simulink library "EmE_MBD_Blockset"  (R2018a)
settings: Solver=ode1  StartTime=0.0  StopTime=Inf  FixedStep=0.001  RelTol=1e-3  EnableMultiTasking=on
PostLoadFcn:
  | , if any(exist('dsrtsu_mdlpostloadfcn', 'file') == [2, 3, 6]), try dsrtsu_mdlpostloadfcn('Execute', bdroot); catch fprintf('Error in PostLoadFcn (dsrtsu_mdlpostloadfcn) for model "%s":\n %s\n', bdroot, lasterr); end, end,
undefined symbols (not defined in the file or in its folder): ENUM_TSC1_CONTROL_PURPOSE_T, gcbh, GLB_SWITCH_T
libraries: simulink x237, $bdroot x115, simulink_need_slupdate x26, MotoHawk_lib x13, simulink_extras x3
(part 3 of 11)

== system EmE_MBD_Blockset/Sources ==
  In : Inport
  APV : Constant  Value=0  mask(Constant APV (EmE)){conval=0}
      mask prompts: conval "Tunable parameter:"
      mask help: Generate a tunable parameter value (configuration or calibration).
      mask init:
      | set_param(gcbh,'Value',conval)
  CPV : Constant  Value=0  mask(Constant CPV (EmE)){conval=0}
      mask prompts: conval "Constant value:"
      mask help: Generate a constant value.
      mask init:
      | set_param(gcbh,'Value',conval)
      mask DialogControl DescTextVar Prompt: Constant parameter value.
  Digital Clock : DigitalClock  SampleTime=-1
  Ground : Ground
  dT : Subsystem  mask(Delta time (dT) (EmE)){}
      mask help: This block calculates a "delta time" or execution rate of a subsystem.
      mask init:
      | alpha=0:2*pi/100:2*pi;
      mask Display:
      | plot(0.3+0.15*cos(alpha),0.5+0.4*sin(alpha));
      | plot([0.3 0.3 0.4],[0.7 0.5 0.5]);
      | fprintf('              dT');

== system EmE_MBD_Blockset/User-Defined Functions ==
  Compare_VIN_data : Subsystem
  Determine_engine_speed_from_vehicle_speed : Subsystem
  Determine_permanent_magnet_motor_BEMF_volts_at_magnet_temp : Subsystem
  Determine_vehicle_speed_from_trans_output_shaft_speed : Subsystem
  Latching_mutual_exclusion : Subsystem
  Snoop : Subsystem  mask(CCP_Snoop){setup=off, a2l=DC4_A1519R191A_modified_checksum.a2l, frstPID=64, sizeDAQ=16, name1=CA_Ambient_air_temp_value, name2=Air_temp_post_int.Value, name3=CPM_Crank_power, name4=CA_Vehicle_speed, name5=CA_Ecfan_fspd_value, name6=CPM_Air_temp_pre_int, name7=AMF_Fresh_air, name8=CA_Ambient_air_press_value, name9=CA_Engine_speed, name10=CA_Cool_temp_value, name11=CREC_Eng_run_time_since_key_on, name12=F_CPM_Int_enabled, address1=400076EC, address2=00501F12, address3=4000C33C, address4=40007564, address5=40007D66, address6=4000C33A, address7=4000BF4A, address8=4000768C, address9=40007530, address10=4000750C, address11=40006210, address12=4000C324, type1=single, type2=uint16, type3=int16, type4=single, type5=uint16, type6=uint16, type7=uint16, type8=single, type9=single, type10=single, type11=uint32, type12=uint8, convert1=[1  1  0], convert2=[1  10   0], convert3=[1  10   0], convert4=[1  1  0], convert5=[1  1  0], convert6=[1  10   0], convert7=[1  40   0], convert8=[1  1  0], convert9=[1  1  0], convert10=[1  1  0], convert11=[1  1  0], convert12=[1  1  0], default1=0, default2=0, default3=0, default4=0, default5=0, default6=0, default7=0, default8=0, default9=0, default10=0, default11=0, default12=0}
      mask prompts: setup "Check to launch auto setup"; a2l "SoftwareA2L"; frstPID "First PID (as dec)"; sizeDAQ "DAQ Length (as dec)"; name1 "Signal Name"; name2 "Signal Name"; name3 "Signal Name"; name4 "Signal Name"; name5 "Signal Name"; name6 "Signal Name"; name7 "Signal Name"; name8 "Signal Name"; name9 "Signal Name"; name10 "Signal Name"; name11 "Signal Name"; name12 "Signal Name"; address1 "Memory Address"; address2 "Memory Address"; address3 "Memory Address"; address4 "Memory Address"; address5 "Memory Address"; address6 "Memory Address"; address7 "Memory Address"; address8 "Memory Address"; address9 "Memory Address"; address10 "Memory Address"; address11 "Memory Address"; address12 "Memory Address"; type1 "Data Type"; type2 "Data Type"; type3 "Data Type"; type4 "Data Type"; type5 "Data Type"; type6 "Data Type"; type7 "Data Type"; type8 "Data Type"; type9 "Data Type"; type10 "Data Type"; type11 "Data Type"; type12 "Data Type"; convert1 "Signal conversion vector [A B C] :: (A/B) * x + C"; convert2 "Signal conversion vector [A B C] :: (A/B) * x + C"; convert3 "Signal conversion vector [A B C] :: (A/B) * x + C"; convert4 "Signal conversion vector [A B C] :: (A/B) * x + C"; convert5 "Signal conversion vector [A B C] :: (A/B) * x + C"; convert6 "Signal conversion vector [A B C] :: (A/B) * x + C"; convert7 "Signal conversion vector [A B C] :: (A/B) * x + C"; convert8 "Signal conversion vector [A B C] :: (A/B) * x + C"; convert9 "Signal conversion vector [A B C] :: (A/B) * x + C"; convert10 "Signal conversion vector [A B C] :: (A/B) * x + C"; convert11 "Signal conversion vector [A B C] :: (A/B) * x + C"; convert12 "Signal conversion vector [A B C] :: (A/B) * x + C"; default1 "Default Value"; default2 "Default Value"; default3 "Default Value"; default4 "Default Value"; default5 "Default Value"; default6 "Default Value"; default7 "Default Value"; default8 "Default Value"; default9 "Default Value"; default10 "Default Value"; default11 "Default Value"; default12 "Default Value"
      mask init:
      | CCP_Snoop_init
      mask Callback setup: snoop_cfg(gcbh)
      mask TypeOptions type1: uint8 | int8 | uint16 | int16 | uint32 | int32 | single
      mask TypeOptions type2: uint8 | int8 | uint16 | int16 | uint32 | int32 | single
      mask TypeOptions type3: uint8 | int8 | uint16 | int16 | uint32 | int32 | single
      mask TypeOptions type4: uint8 | int8 | uint16 | int16 | uint32 | int32 | single
      mask TypeOptions type5: uint8 | int8 | uint16 | int16 | uint32 | int32 | single
      mask TypeOptions type6: uint8 | int8 | uint16 | int16 | uint32 | int32 | single
      mask TypeOptions type7: uint8 | int8 | uint16 | int16 | uint32 | int32 | single
      mask TypeOptions type8: uint8 | int8 | uint16 | int16 | uint32 | int32 | single
      mask TypeOptions type9: uint8 | int8 | uint16 | int16 | uint32 | int32 | single
      mask TypeOptions type10: uint8 | int8 | uint16 | int16 | uint32 | int32 | single
      mask TypeOptions type11: uint8 | int8 | uint16 | int16 | uint32 | int32 | single
      mask TypeOptions type12: uint8 | int8 | uint16 | int16 | uint32 | int32 | single
      mask DialogControl ParameterTabVar0 Prompt: Setup
      mask DialogControl ParameterTabVar01 Prompt: Signal1
      mask DialogControl ParameterTabVar012 Prompt: Signal2
      mask DialogControl ParameterTabVar0123 Prompt: Signal3
      mask DialogControl ParameterTabVar01234 Prompt: Signal4
      mask DialogControl ParameterTabVar012345 Prompt: Signal5
      mask DialogControl ParameterTabVar0123456 Prompt: Signal6
      mask DialogControl ParameterTabVar01234567 Prompt: Signal7
      mask DialogControl ParameterTabVar012345678 Prompt: Signal8
      mask DialogControl ParameterTabVar0123456789 Prompt: Signal9
      mask DialogControl ParameterTabVar012345678910 Prompt: Signal10
      mask DialogControl ParameterTabVar01234567891011 Prompt: Signal11
      mask DialogControl ParameterTabVar0123456789101112 Prompt: Signal12
      mask Display:
      | image(imread('snoop.jpg'))
      | % port_label('output',1,'Data')
      | text(.021,.95,a2lFile,'horizontalAlign', 'left')
      | text(1,0.5,sigDisp,'horizontalAlign', 'right')
  TRUCK_1841_VIN_CPV : Constant  Value=uint8('2NKHHM7X5JM216659')
  wires:
  TRUCK_1841_VIN_CPV/1 -> Compare_VIN_data/1(VIN_Input_uint8)

== system EmE_MBD_Blockset/Controllers/Generic_PID_Governor_3 ==
  F_GPID_reset : Inport
  GPID_setpoint : Inport  Port=2
  GPID_feedback : Inport  Port=3
  GPID_actual_system_output : Inport  Port=4
  GPID_slew_init : Inport  Port=5
  GPID_feed_forward : Inport  Port=6
  GPID_slew_inc_setpoint : Inport  Port=7
  GPID_slew_dec_setpoint : Inport  Port=8
  GPID_output_max : Inport  Port=9
  GPID_output_min : Inport  Port=10
  GPID_Kp : Inport  Port=11
  GPID_Ki : Inport  Port=12
  GPID_Kd : Inport  Port=13
  GPID_T_filt_d : Inport  Port=14
  GPID_T_filt_control_error : Inport  Port=15
  F_GPID_aw_cond_integration : Inport  Port=16
  GPID_aw_hysteresis : Inport  Port=17
  GPID_dT : Inport  Port=18
  F_GPID_aw_hold_i_term : Inport  Port=19
  Calculate_PID_terms : Subsystem
  Determine_control_error : Subsystem
  Output_PID : Subsystem
  Reset_governor : Subsystem
  Unit_Delay : UnitDelay  SampleTime=-1
      settings: AttributesFormatString=IC: %<vinit>
  GPID_output : Outport
  GPID_output_unlim : Outport  Port=2
  GPID_control_error : Outport  Port=3
  GPID_p_term : Outport  Port=4
  GPID_i_term : Outport  Port=5
  GPID_d_term : Outport  Port=6
  F_GPID_hold_i_term : Outport  Port=7
  wires:
  Output_PID/2(GPID_output_unlim) -> GPID_output_unlim/1, Unit_Delay/1
  Calculate_PID_terms/1(GPID_p_term) -> Output_PID/1(GPID_p_term), GPID_p_term/1
  F_GPID_aw_hold_i_term/1 -> Calculate_PID_terms/12(F_GPID_aw_hold_i_term)
  GPID_aw_hysteresis/1 -> Calculate_PID_terms/11(GPID_aw_hysteresis)
  F_GPID_aw_cond_integration/1 -> Calculate_PID_terms/10(F_GPID_aw_cond_integration)
  GPID_feed_forward/1 -> Output_PID/6(GPID_feed_forward), Calculate_PID_terms/5(GPID_feed_forward)
  GPID_actual_system_output/1 -> Calculate_PID_terms/4(GPID_actual_system_output)
  GPID_output_min/1 -> Output_PID/4(GPID_output_min)
  GPID_output_max/1 -> Output_PID/5(GPID_output_max)
  GPID_Kd/1 -> Calculate_PID_terms/8(GPID_Kd)
  GPID_Ki/1 -> Calculate_PID_terms/7(GPID_Ki)
  GPID_feedback/1 -> Determine_control_error/7(GPID_feedback)
  GPID_slew_dec_setpoint/1 -> Determine_control_error/5(GPID_slew_dec_setpoint)
  GPID_setpoint/1 -> Determine_control_error/3(GPID_setpoint)
  GPID_slew_init/1 -> Determine_control_error/2(GPID_slew_init)
  F_GPID_reset/1 -> Reset_governor/1(F_GPID_reset)
  Calculate_PID_terms/4(F_GPID_hold_i_term) -> F_GPID_hold_i_term/1
  Calculate_PID_terms/3(GPID_d_term) -> Output_PID/3(GPID_d_term), GPID_d_term/1
  GPID_T_filt_control_error/1 -> Determine_control_error/8(GPID_T_filt_control_error)
  Reset_governor/1(F_GPID_reset_gov) -> Determine_control_error/1(F_GPID_reset_gov), Calculate_PID_terms/1(F_GPID_reset_gov)
  GPID_slew_inc_setpoint/1 -> Determine_control_error/4(GPID_slew_inc_setpoint)
  GPID_Kp/1 -> Calculate_PID_terms/6(GPID_Kp)
  Determine_control_error/1(GPID_control_error) -> Calculate_PID_terms/2(GPID_control_error), GPID_control_error/1
  Calculate_PID_terms/2(GPID_i_term) -> Output_PID/2(GPID_i_term), GPID_i_term/1
  GPID_T_filt_d/1 -> Calculate_PID_terms/9(GPID_T_filt_d)
  GPID_dT/1 -> Determine_control_error/6(GPID_dT), Calculate_PID_terms/3(GPID_dT)
  Unit_Delay/1 -> Calculate_PID_terms/13(GPID_output_unlim_prev)
  Output_PID/1(GPID_output) -> GPID_output/1

== system EmE_MBD_Blockset/Controllers/Generic_PID_Governor_4 ==
  F_GPID_reset : Inport
  GPID_setpoint : Inport  Port=2
  GPID_feedback : Inport  Port=3
  GPID_actual_system_output : Inport  Port=4
  GPID_slew_init : Inport  Port=5
  GPID_feed_forward : Inport  Port=6
  GPID_slew_inc_setpoint : Inport  Port=7
  GPID_slew_dec_setpoint : Inport  Port=8
  GPID_output_max : Inport  Port=9
  GPID_output_min : Inport  Port=10
  GPID_Kp : Inport  Port=11
  GPID_Ki : Inport  Port=12
  GPID_Kd : Inport  Port=13
  GPID_T_filt_d : Inport  Port=14
  GPID_T_filt_control_error : Inport  Port=15
  F_GPID_aw_cond_integration : Inport  Port=16
  GPID_aw_hysteresis : Inport  Port=17
  GPID_dT : Inport  Port=18
  F_GPID_aw_hold_i_term : Inport  Port=19
  Calculate_PID_terms : Subsystem
  Determine_control_error : Subsystem
  Output_PID : Subsystem
  Reset_governor : Subsystem
  Unit_Delay : UnitDelay  SampleTime=-1
      settings: AttributesFormatString=IC: %<vinit>
  Unit_Delay1 : UnitDelay  SampleTime=-1
      settings: AttributesFormatString=IC: %<vinit>
  GPID_output : Outport
  GPID_output_unlim : Outport  Port=2
  GPID_control_error : Outport  Port=3
  GPID_p_term : Outport  Port=4
  GPID_i_term : Outport  Port=5
  GPID_d_term : Outport  Port=6
  F_GPID_hold_i_term : Outport  Port=7
  wires:
  F_GPID_reset/1 -> Reset_governor/1(F_GPID_reset)
  Reset_governor/1(F_GPID_reset_gov) -> Calculate_PID_terms/1(F_GPID_reset_gov), Determine_control_error/1(F_GPID_reset_gov)
  GPID_slew_init/1 -> Determine_control_error/2(GPID_slew_init)
  GPID_setpoint/1 -> Determine_control_error/3(GPID_setpoint)
  GPID_slew_inc_setpoint/1 -> Determine_control_error/4(GPID_slew_inc_setpoint)
  GPID_slew_dec_setpoint/1 -> Determine_control_error/5(GPID_slew_dec_setpoint)
  GPID_feedback/1 -> Determine_control_error/7(GPID_feedback)
  GPID_T_filt_control_error/1 -> Determine_control_error/8(GPID_T_filt_control_error)
  Determine_control_error/1(GPID_control_error) -> GPID_control_error/1, Calculate_PID_terms/2(GPID_control_error)
  GPID_actual_system_output/1 -> Calculate_PID_terms/4(GPID_actual_system_output)
  GPID_feed_forward/1 -> Output_PID/6(GPID_feed_forward), Calculate_PID_terms/5(GPID_feed_forward)
  GPID_Kp/1 -> Calculate_PID_terms/6(GPID_Kp)
  GPID_Ki/1 -> Calculate_PID_terms/7(GPID_Ki)
  GPID_Kd/1 -> Calculate_PID_terms/8(GPID_Kd)
  GPID_T_filt_d/1 -> Calculate_PID_terms/9(GPID_T_filt_d)
  F_GPID_aw_cond_integration/1 -> Calculate_PID_terms/10(F_GPID_aw_cond_integration)
  GPID_aw_hysteresis/1 -> Calculate_PID_terms/11(GPID_aw_hysteresis)
  GPID_dT/1 -> Determine_control_error/6(GPID_dT), Calculate_PID_terms/3(GPID_dT)
  F_GPID_aw_hold_i_term/1 -> Calculate_PID_terms/12(F_GPID_aw_hold_i_term)
  Calculate_PID_terms/1(GPID_p_term) -> Output_PID/1(GPID_p_term), GPID_p_term/1
  Calculate_PID_terms/2(GPID_i_term) -> Output_PID/2(GPID_i_term), GPID_i_term/1
  Calculate_PID_terms/3(GPID_d_term) -> GPID_d_term/1, Output_PID/3(GPID_d_term)
  Calculate_PID_terms/4(F_GPID_hold_i_term) -> F_GPID_hold_i_term/1
  Unit_Delay/1 -> Calculate_PID_terms/13(GPID_output_unlim_prev)
  GPID_output_max/1 -> Output_PID/5(GPID_output_max)
  GPID_output_min/1 -> Output_PID/4(GPID_output_min)
  Output_PID/1(GPID_output) -> GPID_output/1
  Output_PID/2(GPID_output_unlim) -> GPID_output_unlim/1, Unit_Delay/1
  Unit_Delay1/1 -> Calculate_PID_terms/14(GPID_output_delta)
  Output_PID/3(GPID_output_delta) -> Unit_Delay1/1

== system EmE_MBD_Blockset/Controllers/PID_saturating_terms ==
  Setpoint : Inport
  Feedback : Inport  Port=2
  Feedforward : Inport  Port=3
  Kp : Inport  Port=4
  Ki : Inport  Port=5
  Kd : Inport  Port=6
  Kff : Inport  Port=7
  Kfb : Inport  Port=8
  dT : Inport  Port=9
  P_min : Inport  Port=10
  P_max : Inport  Port=11
  I_min : Inport  Port=12
  I_max : Inport  Port=13
  D_min : Inport  Port=14
  D_max : Inport  Port=15
  Out_min : Inport  Port=16
  Out_max : Inport  Port=17
  Add1 : Sum  Inputs=++++  InputSameDT=on
  Calculate_D_term : Subsystem
  Calculate_I_term : Subsystem
  Calculate_P_term : Subsystem
  Dynamic_saturation3 : $bdroot/Discontinuities/Dynamic_saturation
  Product3 : Product  InputSameDT=on
  Subtract : Sum  Inputs=+-  InputSameDT=on
  Subtract1 : Sum  Inputs=|-+  InputSameDT=on
  Out : Outport
  Out_unlim : Outport  Port=2
  Control_error : Outport  Port=3
  P_term : Outport  Port=4
  I_term : Outport  Port=5
  D_term : Outport  Port=6
  FF_term : Outport  Port=7
  Fb_aw : Outport  Port=8
  wires:
  Setpoint/1 -> Subtract/1
  Feedback/1 -> Subtract/2
  Dynamic_saturation3/1 -> Subtract1/2, Out/1
  Add1/1 -> Subtract1/1, Out_unlim/1, Dynamic_saturation3/2
  Subtract/1 -> Control_error/1, Calculate_D_term/1(Error), Calculate_I_term/1(Error), Calculate_P_term/3(Error)  "error"
  Feedforward/1 -> Product3/1
  Kff/1 -> Product3/2
  Product3/1 -> FF_term/1, Add1/4
  D_max/1 -> Calculate_D_term/2(D_max)
  Kd/1 -> Calculate_D_term/3(Kd)
  D_min/1 -> Calculate_D_term/4(D_min)
  Calculate_D_term/1(Out) -> D_term/1, Add1/3  "d_term"
  Kp/1 -> Calculate_P_term/2(Kp)
  P_min/1 -> Calculate_P_term/4(P_min)
  Calculate_P_term/1(Out) -> P_term/1, Add1/1  "p_term"
  Subtract1/1 -> Calculate_I_term/2(Output_fb_delta)
  dT/1 -> Calculate_D_term/5(dT), Calculate_I_term/3(dT)
  I_max/1 -> Calculate_I_term/4(I_max)
  Ki/1 -> Calculate_I_term/5(Ki)
  I_min/1 -> Calculate_I_term/6(I_min)
  Kfb/1 -> Calculate_I_term/7(K_fb_delta)
  Calculate_I_term/1(Out) -> I_term/1, Add1/2  "i_term"
  Out_max/1 -> Dynamic_saturation3/1
  Out_min/1 -> Dynamic_saturation3/3
  P_max/1 -> Calculate_P_term/1(P_max)
  Calculate_I_term/2(Fb_aw) -> Fb_aw/1

== system EmE_MBD_Blockset/Discontinuities/Debounce ==
  In : Inport
  On_T : Inport  Port=2
  Off_T : Inport  Port=3
  Data Type Conversion : DataTypeConversion  OutDataTypeStr=boolean
      settings: AttributesFormatString=%<OutDataTypeStr>
  Debounce_state_machine : Stateflow chart  Tag=Chart_v1  TreatAsAtomicUnit=on
  Debounce_timers : Subsystem
  Out : Outport  OutputWhenDisabled=reset
  wires:
  In/1 -> Data Type Conversion/1
  Data Type Conversion/1 -> Debounce_timers/1(F_In), Debounce_state_machine/1(F_In)
  Debounce_timers/1(F_On_timer_complete) -> Debounce_state_machine/2(F_On_timer_complete)
  Debounce_timers/2(F_Off_timer_complete) -> Debounce_state_machine/3(F_Off_timer_complete)
  On_T/1 -> Debounce_timers/2(On_timer_T_secs)
  Off_T/1 -> Debounce_timers/3(Off_timer_T_secs)
  Debounce_state_machine/1(F_Out) -> Out/1

== system EmE_MBD_Blockset/Discontinuities/Dynamic_saturation ==
  Max : Inport
  In : Inport  Port=2
  Min : Inport  Port=3
  If_Then_Else : $bdroot/Signal Routing/If_Then_Else
  If_Then_Else1 : $bdroot/Signal Routing/If_Then_Else
  Relational Operator : RelationalOperator  Operator=<=  OutDataTypeStr=boolean  RndMeth=Nearest  InputSameDT=on
  Relational Operator1 : RelationalOperator  OutDataTypeStr=boolean  RndMeth=Nearest  InputSameDT=on
  Out : Outport
  wires:
  Max/1 -> Relational Operator1/2, If_Then_Else/2
  Relational Operator/1 -> If_Then_Else1/1
  If_Then_Else/1 -> Out/1
  Relational Operator1/1 -> If_Then_Else/1
  Min/1 -> Relational Operator/2, If_Then_Else1/2
  In/1 -> If_Then_Else1/3, Relational Operator/1, Relational Operator1/1
  If_Then_Else1/1 -> If_Then_Else/3

== system EmE_MBD_Blockset/Discontinuities/Falling_edge ==
  In : Inport  OutDataTypeStr=boolean
  Logical Operator : Logic  OutDataTypeStr=boolean
  Logical Operator1 : Logic  Operator=NOT  OutDataTypeStr=boolean
  Unit_Delay : UnitDelay  InitialCondition=false  SampleTime=-1
      settings: AttributesFormatString=IC: %<InitialCondition>
  Out : Outport  OutDataTypeStr=boolean
  wires:
  Logical Operator/1 -> Out/1
  In/1 -> Unit_Delay/1, Logical Operator1/1
  Unit_Delay/1 -> Logical Operator/1
  Logical Operator1/1 -> Logical Operator/2

== system EmE_MBD_Blockset/Discontinuities/Hysteresis ==
  High : Inport
  In : Inport  Port=2
  Low : Inport  Port=3
  Constant : Constant  Value=true
  Constant1 : Constant  Value=false
  If_Then_Else : $bdroot/Signal Routing/If_Then_Else
  If_Then_Else1 : $bdroot/Signal Routing/If_Then_Else
  Relational Operator : RelationalOperator  Operator=<=  OutDataTypeStr=boolean  RndMeth=Nearest  InputSameDT=on
  Relational Operator1 : RelationalOperator  OutDataTypeStr=boolean  RndMeth=Nearest  InputSameDT=on
  Unit_Delay : UnitDelay  InitialCondition=false  SampleTime=-1
      settings: AttributesFormatString=IC: %<InitialCondition>
  Out : Outport  OutDataTypeStr=boolean
  wires:
  High/1 -> Relational Operator1/2
  Unit_Delay/1 -> If_Then_Else1/3
  Relational Operator1/1 -> If_Then_Else/1
  If_Then_Else1/1 -> If_Then_Else/3
  Constant1/1 -> If_Then_Else1/2
  Constant/1 -> If_Then_Else/2
  If_Then_Else/1 -> Out/1, Unit_Delay/1
  Low/1 -> Relational Operator/2
  Relational Operator/1 -> If_Then_Else1/1
  In/1 -> Relational Operator1/1, Relational Operator/1

== system EmE_MBD_Blockset/Discontinuities/Rising_edge ==
  In : Inport  OutDataTypeStr=boolean
  Logical Operator : Logic  OutDataTypeStr=boolean
  Logical Operator1 : Logic  Operator=NOT  OutDataTypeStr=boolean
  Unit_Delay : UnitDelay  InitialCondition=true  SampleTime=-1
      settings: AttributesFormatString=IC: %<InitialCondition>
  Out : Outport  OutDataTypeStr=boolean
  wires:
  Logical Operator/1 -> Out/1
  Unit_Delay/1 -> Logical Operator1/1
  In/1 -> Logical Operator/1, Unit_Delay/1
  Logical Operator1/1 -> Logical Operator/2

== system EmE_MBD_Blockset/Discrete/DT1_Derivative_lag ==
  F_Reset : Inport
  In : Inport  Port=2
  Init : Inport  Port=3
  T : Inport  Port=4
  dT : Inport  Port=5
  K : Inport  Port=6
  Add1 : Sum  InputSameDT=on
  Constant : Constant  Value=false
  Constant1 : Constant  Value=-1
  Cubic_Approximation : Subsystem
  Divide : Product  Inputs=*/  InputSameDT=on
  If_Then_Else : $bdroot/Signal Routing/If_Then_Else
  Logical Operator : Logic  Operator=OR  OutDataTypeStr=boolean
  MinMax1 : MinMax  Function=max  Inputs=2  InputSameDT=on
  Product1 : Product  InputSameDT=on
  Product2 : Product  InputSameDT=on
  Product3 : Product  InputSameDT=on
  Subtract1 : Sum  Inputs=+-  InputSameDT=on
  Unit_Delay1 : UnitDelay  InitialCondition=true  SampleTime=-1
      settings: AttributesFormatString=IC: %<vinit>
  Unit_Delay2 : UnitDelay  SampleTime=-1
      settings: AttributesFormatString=IC: %<vinit>
  Unit_Delay3 : UnitDelay  SampleTime=-1
      settings: AttributesFormatString=IC: %<vinit>
  Out : Outport
  wires:
  Add1/1 -> Product1/2
  Cubic_Approximation/1(Out1) -> Product1/1
  Divide/1 -> Product2/1
  Constant/1 -> Unit_Delay1/1
  Logical Operator/1 -> If_Then_Else/1
  Unit_Delay1/1 -> Logical Operator/2
  Init/1 -> If_Then_Else/2
  F_Reset/1 -> Logical Operator/1
  If_Then_Else/1 -> Out/1, Unit_Delay2/1
  T/1 -> MinMax1/2
  MinMax1/1 -> Divide/2
  dT/1 -> MinMax1/1, Divide/1
  Constant1/1 -> Product2/2
  In/1 -> Subtract1/1, Unit_Delay3/1
  Unit_Delay3/1 -> Subtract1/2
  Product2/1 -> Cubic_Approximation/1(In1)
  Unit_Delay2/1 -> Add1/2
  Product1/1 -> If_Then_Else/3
  Product3/1 -> Add1/1
  K/1 -> Product3/1
  Subtract1/1 -> Product3/2

== system EmE_MBD_Blockset/Discrete/Discrete Derivative ==
  In : Inport
  IC : Inport  Port=2
  K : Inport  Port=3
  dT : Inport  Port=4
  Divide1 : Product  Inputs=**/  InputSameDT=on
  Subtract1 : Sum  Inputs=+-  InputSameDT=on
  Unit Delay External IC : simulink_need_slupdate/Unit Delay External IC  tsamp=-1
      settings: SourceProductName=Simulink  SourceProductBaseCode=SL
  Out : Outport  LibraryBlock=$bdroot/Sinks/Out  OutputWhenDisabled=reset
  wires:
  Unit Delay External IC/1 -> Subtract1/2
  In/1 -> Divide1/1
  Divide1/1 -> Subtract1/1, Unit Delay External IC/1
  Subtract1/1 -> Out/1
  IC/1 -> Unit Delay External IC/2
  K/1 -> Divide1/2
  dT/1 -> Divide1/3

== system EmE_MBD_Blockset/Discrete/Discrete-Time Integrator ==
  F_Reset : Inport
  U : Inport  Port=2
  K : Inport  Port=3
  dT : Inport  Port=4
  Add : Sum  InputSameDT=on
  CPV : $bdroot/Sources/CPV  conval=0
  Integrator_method : Subsystem
  Product1 : Product  Inputs=3  InputSameDT=on
  Unit Delay Resettable External IC1 : simulink_need_slupdate/Unit Delay Resettable External IC  tsamp=-1
      settings: SourceProductName=Simulink  SourceProductBaseCode=SL
  Y : Outport  OutputWhenDisabled=reset  InitialOutput=0
  wires:
  K/1 -> Product1/1
  Unit Delay Resettable External IC1/1 -> Add/1
  Add/1 -> Unit Delay Resettable External IC1/1, Y/1
  CPV/1 -> Unit Delay Resettable External IC1/3
  Product1/1 -> Add/2
  F_Reset/1 -> Unit Delay Resettable External IC1/2, Integrator_method/2(F_Reset)
  Integrator_method/1(U_out) -> Product1/2
  U/1 -> Integrator_method/1(U_in)
  dT/1 -> Product1/3

== system EmE_MBD_Blockset/Discrete/Exponential_weighted_average ==
  F_Enable : Inport
  F_Reset : Inport  Port=2
  In : Inport  Port=3
  K : Inport  Port=4
  Add : Sum  InputSameDT=on
  Add1 : Sum  InputSameDT=on
  Constant : Constant
  Constant1 : Constant
  Constant2 : Constant  Value=0.001
  Constant3 : Constant
  Divide : Product  Inputs=*/  InputSameDT=on
  Dynamic_saturation : $bdroot/Discontinuities/Dynamic_saturation
  If_Then_Else : $bdroot/Signal Routing/If_Then_Else
  If_Then_Else1 : $bdroot/Signal Routing/If_Then_Else
  Product : Product  InputSameDT=on
  Product1 : Product  InputSameDT=on
  Product2 : Product  InputSameDT=on
  Subtract : Sum  Inputs=+-  InputSameDT=on
  Unit Delay Resettable External IC : simulink_need_slupdate/Unit Delay Resettable External IC  tsamp=-1
      settings: SourceProductName=Simulink  SourceProductBaseCode=SL
  Unit Delay Resettable External IC1 : simulink_need_slupdate/Unit Delay Resettable External IC  tsamp=-1
      settings: SourceProductName=Simulink  SourceProductBaseCode=SL
  Out : Outport
  wires:
  Add/1 -> If_Then_Else1/2
  If_Then_Else/1 -> Out/1, Unit Delay Resettable External IC1/3, Unit Delay Resettable External IC1/1
  In/1 -> Product2/2
  K/1 -> Dynamic_saturation/2
  Product/1 -> Add/1
  F_Reset/1 -> Unit Delay Resettable External IC1/2, Unit Delay Resettable External IC/2
  Constant/1 -> Unit Delay Resettable External IC/3, Add/2
  Constant1/1 -> Subtract/1, Divide/1
  Divide/1 -> Subtract/2, Product2/1
  Subtract/1 -> Product1/1
  Product1/1 -> Add1/1
  Product2/1 -> Add1/2
  Unit Delay Resettable External IC1/1 -> Product1/2, If_Then_Else/3
  F_Enable/1 -> If_Then_Else1/1, If_Then_Else/1
  Dynamic_saturation/1 -> Product/1
  Constant2/1 -> Dynamic_saturation/3
  Constant3/1 -> Dynamic_saturation/1
  Add1/1 -> If_Then_Else/2
  Unit Delay Resettable External IC/1 -> Divide/2, If_Then_Else1/3, Product/2
  If_Then_Else1/1 -> Unit Delay Resettable External IC/1

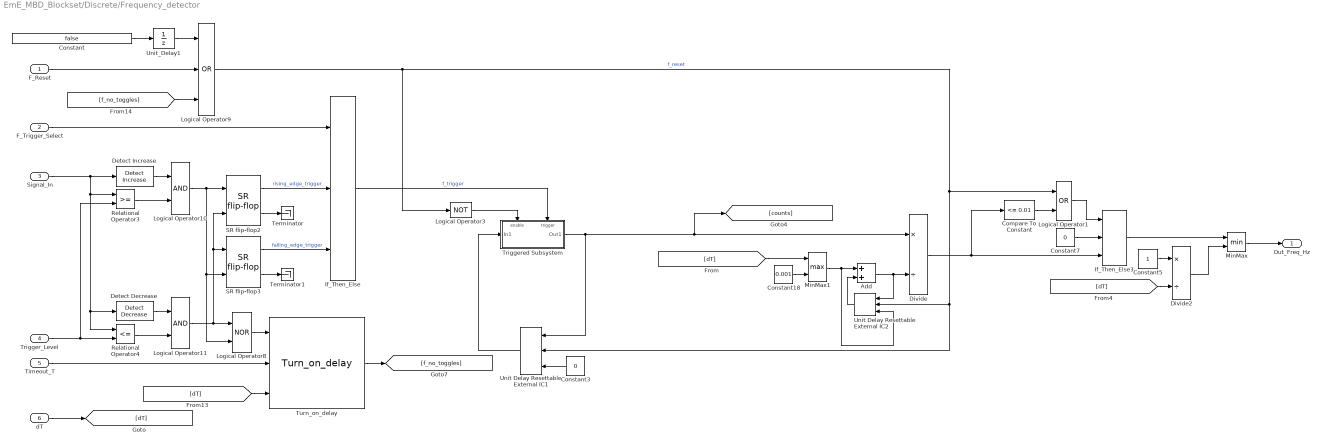
== system EmE_MBD_Blockset/Discrete/Frequency_detector ==
  F_Reset : Inport
  F_Trigger_Select : Inport  Port=2
  Signal_In : Inport  Port=3
  Trigger_Level : Inport  Port=4
  Timeout_T : Inport  Port=5
  dT : Inport  Port=6
  Add : Sum
  Compare To Constant : simulink/Logic and Bit Operations/Compare To Constant  relop=<=  const=0.01  OutDataTypeStr=boolean
  Constant : Constant  Value=false
  Constant18 : Constant  Value=0.001
  Constant3 : Constant  Value=0
  Constant5 : Constant
  Constant7 : Constant  Value=0
  Detect Decrease : simulink/Logic and Bit Operations/Detect Decrease  vinit=0  InputProcessing=Inherited  OutDataTypeStr=boolean
  Detect Increase : simulink/Logic and Bit Operations/Detect Increase  vinit=0  InputProcessing=Inherited  OutDataTypeStr=boolean
  Divide : Product  Inputs=*/
  Divide2 : Product  Inputs=*/
  If_Then_Else : $bdroot/Signal Routing/If_Then_Else
  If_Then_Else3 : $bdroot/Signal Routing/If_Then_Else
  Logical Operator1 : Logic  Operator=OR  AllPortsSameDT=off  OutDataTypeStr=boolean
  Logical Operator10 : Logic  OutDataTypeStr=boolean
  Logical Operator11 : Logic  OutDataTypeStr=boolean
  Logical Operator3 : Logic  Operator=NOT  OutDataTypeStr=boolean
  Logical Operator8 : Logic  Operator=NOR  AllPortsSameDT=off  OutDataTypeStr=boolean
  Logical Operator9 : Logic  Operator=OR  Inputs=3  OutDataTypeStr=boolean
  MinMax : MinMax  Inputs=2
  MinMax1 : MinMax  Function=max  Inputs=2
  Relational Operator3 : RelationalOperator  OutDataTypeStr=boolean  RndMeth=Nearest  InputSameDT=on
  Relational Operator4 : RelationalOperator  Operator=<=  OutDataTypeStr=boolean  RndMeth=Nearest  InputSameDT=on
  SR flip-flop2 : $bdroot/Logic and Bit Operations/SR flip-flop
  SR flip-flop3 : $bdroot/Logic and Bit Operations/SR flip-flop
  Terminator : Terminator
  Terminator1 : Terminator
  Triggered Subsystem : Subsystem  TreatAsAtomicUnit=on
  Turn_on_delay : $bdroot/Discrete/Turn_on_delay
  Unit Delay Resettable External IC1 : simulink_need_slupdate/Unit Delay Resettable External IC  tsamp=-1
      settings: SourceProductName=Simulink  SourceProductBaseCode=SL
  Unit Delay Resettable External IC2 : simulink_need_slupdate/Unit Delay Resettable External IC  tsamp=-1
      settings: SourceProductName=Simulink  SourceProductBaseCode=SL
  Unit_Delay1 : UnitDelay  InitialCondition=true  SampleTime=-1
      settings: AttributesFormatString=IC: %<vinit>
  Out_Freq_Hz : Outport
  wires:
  Unit_Delay1/1 -> Logical Operator9/1
  dT/1 -> [dT]
  If_Then_Else3/1 -> MinMax/1
  MinMax/1 -> Out_Freq_Hz/1
  Logical Operator3/1 -> Triggered Subsystem/Enable
  Constant7/1 -> If_Then_Else3/2
  Constant18/1 -> MinMax1/2
  Divide/1 -> If_Then_Else3/3, Compare To Constant/1
  Constant3/1 -> Unit Delay Resettable External IC1/3
  Compare To Constant/1 -> Logical Operator1/2
  Triggered Subsystem/1(Out1) -> Divide/1, [counts], Unit Delay Resettable External IC1/1
  Logical Operator9/1 -> Unit Delay Resettable External IC1/2, Unit Delay Resettable External IC2/2, Logical Operator1/1, Logical Operator3/1  "f_reset"
  [dT] -> Divide2/2
  Add/1 -> Unit Delay Resettable External IC2/1, Divide/2
  Logical Operator1/1 -> If_Then_Else3/1
  If_Then_Else/1 -> Triggered Subsystem/Trigger  "f_trigger"
  [f_no_toggles] -> Logical Operator9/3
  [dT] -> MinMax1/1
  Constant5/1 -> Divide2/1
  MinMax1/1 -> Unit Delay Resettable External IC2/3, Add/1
  Unit Delay Resettable External IC1/1 -> Triggered Subsystem/1(In1)
  Divide2/1 -> MinMax/2
  Unit Delay Resettable External IC2/1 -> Add/2
  F_Reset/1 -> Logical Operator9/2
  Constant/1 -> Unit_Delay1/1
  SR flip-flop3/1 -> If_Then_Else/3  "falling_edge_trigger"
  Logical Operator11/1 -> SR flip-flop2/2, SR flip-flop3/1, Logical Operator8/1
  Relational Operator3/1 -> Logical Operator10/2
  Trigger_Level/1 -> Relational Operator4/2, Relational Operator3/2
  Relational Operator4/1 -> Logical Operator11/2
  F_Trigger_Select/1 -> If_Then_Else/1
  SR flip-flop3/2 -> Terminator1/1
  SR flip-flop2/1 -> If_Then_Else/2  "rising_edge_trigger"
  Detect Decrease/1 -> Logical Operator11/1
  Logical Operator8/1 -> Turn_on_delay/1
  Logical Operator10/1 -> SR flip-flop2/1, SR flip-flop3/2, Logical Operator8/2
  Signal_In/1 -> Relational Operator4/1, Detect Decrease/1, Relational Operator3/1, Detect Increase/1
  SR flip-flop2/2 -> Terminator/1
  Detect Increase/1 -> Logical Operator10/1
  Turn_on_delay/1 -> [f_no_toggles]
  Timeout_T/1 -> Turn_on_delay/2
  [dT] -> Turn_on_delay/3

== system EmE_MBD_Blockset/Discrete/LPF_first_order ==
  F_Reset : Inport
  In : Inport  Port=2
  Init : Inport  Port=3
  T : Inport  Port=4
  dT : Inport  Port=5
  Add1 : Sum  InputSameDT=on
  Constant : Constant  Value=false
  Constant1 : Constant
  Divide : Product  Inputs=*/  InputSameDT=on
  If_Then_Else : $bdroot/Signal Routing/If_Then_Else
  Logical Operator : Logic  Operator=OR  OutDataTypeStr=boolean
  MinMax1 : MinMax  Function=max  Inputs=2  InputSameDT=on
  Product1 : Product  InputSameDT=on
  Product2 : Product  InputSameDT=on
  Saturation : Saturate  UpperLimit=Inf  LowerLimit=0.0001
  Subtract1 : Sum  Inputs=-+  InputSameDT=on
  Unit_Delay1 : UnitDelay  InitialCondition=true  SampleTime=-1
      settings: AttributesFormatString=IC: %<vinit>
  Unit_Delay2 : UnitDelay  SampleTime=-1
      settings: AttributesFormatString=IC: %<vinit>
  Out : Outport
  wires:
  Constant1/1 -> Subtract1/2
  Divide/1 -> Subtract1/1, Product2/2
  Add1/1 -> If_Then_Else/3
  dT/1 -> MinMax1/1, Divide/1
  T/1 -> MinMax1/2
  Subtract1/1 -> Product1/1
  MinMax1/1 -> Saturation/1
  Unit_Delay2/1 -> Product1/2
  Product2/1 -> Add1/1
  Product1/1 -> Add1/2
  Init/1 -> If_Then_Else/2
  If_Then_Else/1 -> Out/1, Unit_Delay2/1
  Logical Operator/1 -> If_Then_Else/1
  In/1 -> Product2/1
  F_Reset/1 -> Logical Operator/1
  Constant/1 -> Unit_Delay1/1
  Unit_Delay1/1 -> Logical Operator/2
  Saturation/1 -> Divide/2

== system EmE_MBD_Blockset/Discrete/One_shot_pulse ==
  In : Inport
  Duration : Inport  Port=2
  dT : Inport  Port=3
  Add : Sum  InputSameDT=on
  Constant : Constant  Value=false
  Constant1 : Constant  Value=0
  If_Then_Else1 : $bdroot/Signal Routing/If_Then_Else
  If_Then_Else2 : $bdroot/Signal Routing/If_Then_Else
  Relational Operator : RelationalOperator  OutDataTypeStr=boolean  RndMeth=Nearest  InputSameDT=on
  Relational Operator1 : RelationalOperator  Operator=<  OutDataTypeStr=boolean  RndMeth=Nearest  InputSameDT=on
  Rising_edge1 : $bdroot/Discontinuities/Rising_edge  initact=off
      settings: AttributesFormatString=Action on IC: %<initact>
  SR flip-flop1 : $bdroot/Logic and Bit Operations/SR flip-flop
  Terminator : Terminator
  Unit_Delay1 : UnitDelay  SampleTime=-1
      settings: AttributesFormatString=IC: %<vinit>
  Unit_Delay2 : UnitDelay  InitialCondition=false  SampleTime=-1
      settings: AttributesFormatString=IC: %<vinit>
  Out : Outport
  wires:
  If_Then_Else2/1 -> Unit_Delay1/1, Relational Operator/1
  Constant/1 -> If_Then_Else1/2
  If_Then_Else1/1 -> Out/1
  Unit_Delay2/1 -> SR flip-flop1/2
  Rising_edge1/1 -> SR flip-flop1/1
  Constant1/1 -> If_Then_Else2/3
  Relational Operator/1 -> Unit_Delay2/1
  Relational Operator1/1 -> If_Then_Else1/1
  SR flip-flop1/1 -> If_Then_Else1/3, If_Then_Else2/1
  Unit_Delay1/1 -> Add/2
  In/1 -> Rising_edge1/1
  Add/1 -> If_Then_Else2/2
  SR flip-flop1/2 -> Terminator/1
  dT/1 -> Relational Operator1/2, Add/1
  Duration/1 -> Relational Operator/2, Relational Operator1/1

== system EmE_MBD_Blockset/Discrete/PT1_First_order_lag ==
  F_Reset : Inport
  In : Inport  Port=2
  Init : Inport  Port=3
  T : Inport  Port=4
  dT : Inport  Port=5
  K : Inport  Port=6
  Add2 : Sum  InputSameDT=on
  Constant : Constant  Value=false
  Constant1 : Constant  Value=-1
  Constant2 : Constant
  Cubic_Approximation : Subsystem
  Divide : Product  Inputs=*/  InputSameDT=on
  If_Then_Else : $bdroot/Signal Routing/If_Then_Else
  Logical Operator : Logic  Operator=OR  OutDataTypeStr=boolean
  MinMax1 : MinMax  Function=max  Inputs=2  InputSameDT=on
  Product1 : Product  InputSameDT=on
  Product2 : Product  InputSameDT=on
  Product5 : Product  Inputs=3  InputSameDT=on
  Subtract2 : Sum  Inputs=+-  InputSameDT=on
  Unit_Delay1 : UnitDelay  InitialCondition=true  SampleTime=-1
      settings: AttributesFormatString=IC: %<vinit>
  Unit_Delay2 : UnitDelay  SampleTime=-1
      settings: AttributesFormatString=IC: %<vinit>
  Out : Outport
  wires:
  Logical Operator/1 -> If_Then_Else/1
  Constant/1 -> Unit_Delay1/1
  Divide/1 -> Product2/1
  Unit_Delay1/1 -> Logical Operator/2
  F_Reset/1 -> Logical Operator/1
  If_Then_Else/1 -> Out/1, Unit_Delay2/1
  T/1 -> MinMax1/2
  MinMax1/1 -> Divide/2
  Init/1 -> If_Then_Else/2
  dT/1 -> MinMax1/1, Divide/1
  Constant1/1 -> Product2/2
  Product2/1 -> Cubic_Approximation/1(In1)
  Cubic_Approximation/1(Out1) -> Product1/1, Subtract2/2
  Constant2/1 -> Subtract2/1
  Subtract2/1 -> Product5/3
  K/1 -> Product5/1
  In/1 -> Product5/2
  Product5/1 -> Add2/1
  Product1/1 -> Add2/2
  Unit_Delay2/1 -> Product1/2
  Add2/1 -> If_Then_Else/3

== system EmE_MBD_Blockset/Discrete/Savitzky-Golay_Diff_Filter ==
  In : Inport
  Add : Sum  InputSameDT=on
  Add1 : Sum  Inputs=++--  InputSameDT=on
  Constant : Constant  Value=0.1
  Constant1 : Constant  Value=10
  Constant2 : Constant  Value=0.1
  Product{,1..4} (5 alike) : Product  InputSameDT=on
  Unit_Delay{1..4} (4 alike) : UnitDelay  SampleTime=-1
      settings: AttributesFormatString=IC: %<vinit>
  Out : Outport
  wires:
  Product/1 -> Add1/1
  Constant/1 -> Add/1
  Product2/1 -> Add1/2
  Constant1/1 -> Product1/2
  Unit_Delay1/1 -> Unit_Delay2/1, Product2/1
  Product1/1 -> Out/1
  In/1 -> Unit_Delay1/1, Product/1
  Add1/1 -> Product1/1
  Constant2/1 -> Add/2, Product3/1, Product2/2
  Unit_Delay3/1 -> Product3/2, Unit_Delay4/1
  Unit_Delay4/1 -> Product4/2
  Add/1 -> Product4/1, Product/2
  Unit_Delay2/1 -> Unit_Delay3/1
  Product3/1 -> Add1/3
  Product4/1 -> Add1/4

== system EmE_MBD_Blockset/Discrete/Sliding_window_average ==
  F_Enable : Inport
  F_Reset : Inport  Port=2
  Init : Inport  Port=3
  In : Inport  Port=4
  Add : Sum  Inputs=+  InputSameDT=on
  CPV2 : $bdroot/Sources/CPV  conval=false
  Constant : Constant  Value=ones(1,4)
  Demux : Demux  Outputs=[-1 1]
  Divide1 : Product  Inputs=*/  InputSameDT=on
  If_Then_Else{,1..3} (4 alike) : $bdroot/Signal Routing/If_Then_Else
  Logical Operator : $bdroot/Logic and Bit Operations/Logical Operator  Operator=OR  Inputs=2
  Mux : Mux  Inputs=2
  Product : Product  InputSameDT=on
  Terminator : Terminator
  Unit Delay External IC : simulink_need_slupdate/Unit Delay External IC  tsamp=-1
      settings: SourceProductName=Simulink  SourceProductBaseCode=SL
  Unit Delay External IC1 : simulink_need_slupdate/Unit Delay External IC  tsamp=-1
      settings: SourceProductName=Simulink  SourceProductBaseCode=SL
  Unit_Delay : UnitDelay  InitialCondition=true  SampleTime=-1
      settings: AttributesFormatString=IC: %<vinit>
  Width : Width  OutDataTypeMode=All ports same datatype
  Out : Outport
  wires:
  If_Then_Else/1 -> If_Then_Else2/3
  F_Enable/1 -> If_Then_Else1/1, If_Then_Else/1
  Logical Operator/1 -> If_Then_Else3/1, If_Then_Else2/1
  If_Then_Else2/1 -> Unit Delay External IC1/1
  Divide1/1 -> If_Then_Else1/2
  Product/1 -> If_Then_Else2/2
  If_Then_Else3/1 -> Unit Delay External IC/1, Out/1
  If_Then_Else1/1 -> If_Then_Else3/3
  Unit Delay External IC/1 -> If_Then_Else1/3
  Demux/2 -> Terminator/1
  Init/1 -> Product/1, If_Then_Else3/2
  Mux/1 -> Demux/1
  Unit Delay External IC1/1 -> If_Then_Else/3, Mux/2
  In/1 -> Unit Delay External IC/2, Unit Delay External IC1/2, Mux/1
  Add/1 -> Divide1/1
  Demux/1 -> Add/1, If_Then_Else/2
  Width/1 -> Divide1/2
  Constant/1 -> Product/2, Width/1
  CPV2/1 -> Unit_Delay/1
  Unit_Delay/1 -> Logical Operator/2
  F_Reset/1 -> Logical Operator/1

== system EmE_MBD_Blockset/Discrete/Timer_enabled_with_reset ==
  F_Enable : Inport
  F_Reset : Inport  Port=2
  T_init : Inport  Port=3
  T_max : Inport  Port=4
  dT : Inport  Port=5
  Add : Sum  InputSameDT=on
  If_Then_Else1 : $bdroot/Signal Routing/If_Then_Else
  Logical Operator : Logic  OutDataTypeStr=boolean
  Logical Operator1 : Logic  Operator=NOT  OutDataTypeStr=boolean
  MinMax : MinMax  Inputs=2  InputSameDT=on
  Subtract : Sum  Inputs=+-  InputSameDT=on
  Unit Delay Resettable External IC1 : simulink_need_slupdate/Unit Delay Resettable External IC  tsamp=-1
      settings: SourceProductName=Simulink  SourceProductBaseCode=SL
  T_actual : Outport
      settings: AttributesFormatString=IC: %<InitialOutput>\nDisabled value: %<OutputWhenDisabled>
  T_remaining : Outport  Port=2
      settings: AttributesFormatString=IC: %<InitialOutput>\nDisabled value: %<OutputWhenDisabled>
  wires:
  F_Reset/1 -> Unit Delay Resettable External IC1/2, Logical Operator1/1
  MinMax/1 -> If_Then_Else1/2
  T_init/1 -> Unit Delay Resettable External IC1/3
  F_Enable/1 -> Logical Operator/1
  If_Then_Else1/1 -> T_actual/1, Unit Delay Resettable External IC1/1, Subtract/2
  Unit Delay Resettable External IC1/1 -> If_Then_Else1/3, Add/2
  Subtract/1 -> T_remaining/1
  Add/1 -> MinMax/2
  T_max/1 -> MinMax/1, Subtract/1
  Logical Operator/1 -> If_Then_Else1/1
  Logical Operator1/1 -> Logical Operator/2
  dT/1 -> Add/1

== system EmE_MBD_Blockset/Discrete/Turn_off_delay ==
  In : Inport
  Duration : Inport  Port=2
  dT : Inport  Port=3
  Add : Sum  InputSameDT=on
  Constant : Constant  Value=0
  If_Then_Else2 : $bdroot/Signal Routing/If_Then_Else
  If_Then_Else3 : $bdroot/Signal Routing/If_Then_Else
  Logical Operator : Logic  AllPortsSameDT=off  OutDataTypeStr=boolean
  Logical Operator1 : Logic  Operator=NOT  AllPortsSameDT=off  OutDataTypeStr=boolean
  Relational Operator : RelationalOperator  OutDataTypeStr=boolean  RndMeth=Nearest  InputSameDT=on
  Relational Operator1 : RelationalOperator  Operator=<  OutDataTypeStr=boolean  RndMeth=Nearest  InputSameDT=on
  SR flip-flop1 : Subsystem  mask(SR flip-flop (EmE)){}
      mask help: SR flip-flop with priority on set input.
      mask Help:
      | Truth table:<font face="courier">
      | S R Q !Q
      | 0 0 Q !Q
      | 0 1 0  1
      | 1 0 1  0
      | 1 1 1  0
      | </font>
  Terminator : Terminator
  Unit_Delay1 : UnitDelay  SampleTime=-1
      settings: AttributesFormatString=IC: %<vinit>
  Unit_Delay2 : UnitDelay  InitialCondition=false  SampleTime=-1
      settings: AttributesFormatString=IC: %<vinit>
  Out : Outport
  wires:
  Logical Operator/1 -> If_Then_Else2/1
  Relational Operator1/1 -> If_Then_Else3/1
  Unit_Delay2/1 -> SR flip-flop1/2(R)
  If_Then_Else2/1 -> Unit_Delay1/1, Relational Operator/1
  Logical Operator1/1 -> Logical Operator/2
  If_Then_Else3/1 -> Out/1
  Add/1 -> If_Then_Else2/2
  Duration/1 -> Relational Operator/2, Relational Operator1/1
  Relational Operator/1 -> Unit_Delay2/1
  Constant/1 -> If_Then_Else2/3
  Unit_Delay1/1 -> Add/2
  In/1 -> If_Then_Else3/2, SR flip-flop1/1(Sp), Logical Operator1/1
  dT/1 -> Add/1, Relational Operator1/2
  SR flip-flop1/2(!Q) -> Terminator/1
  SR flip-flop1/1(Q) -> If_Then_Else3/3, Logical Operator/1

== system EmE_MBD_Blockset/Discrete/Turn_on_delay ==
  In : Inport
  Duration : Inport  Port=2
  dT : Inport  Port=3
  Add1 : Sum  InputSameDT=on
  Constant1 : Constant  Value=0
  If_Then_Else : $bdroot/Signal Routing/If_Then_Else
  If_Then_Else1 : $bdroot/Signal Routing/If_Then_Else
  Logical Operator2 : Logic  AllPortsSameDT=off  OutDataTypeStr=boolean
  Logical Operator3 : Logic  Operator=NOT  AllPortsSameDT=off  OutDataTypeStr=boolean
  RS flip-flop1 : $bdroot/Logic and Bit Operations/RS flip-flop
  Relational Operator2 : RelationalOperator  OutDataTypeStr=boolean  RndMeth=Nearest  InputSameDT=on
  Relational Operator3 : RelationalOperator  Operator=<  OutDataTypeStr=boolean  RndMeth=Nearest  InputSameDT=on
  Unit_Delay3 : UnitDelay  SampleTime=-1
      settings: AttributesFormatString=IC: %<vinit>
  Unit_Delay4 : UnitDelay  InitialCondition=false  SampleTime=-1
      settings: AttributesFormatString=IC: %<vinit>
  Out : Outport
  wires:
  RS flip-flop1/1 -> If_Then_Else1/3
  Logical Operator2/1 -> If_Then_Else/1
  Duration/1 -> Relational Operator2/2, Relational Operator3/1
  Relational Operator2/1 -> Unit_Delay4/1
  If_Then_Else1/1 -> Out/1
  Constant1/1 -> If_Then_Else/3
  Relational Operator3/1 -> If_Then_Else1/1
  If_Then_Else/1 -> Unit_Delay3/1, Relational Operator2/1
  dT/1 -> Add1/1, Relational Operator3/2
  In/1 -> If_Then_Else1/2, Logical Operator2/2, Logical Operator3/1
  Unit_Delay4/1 -> RS flip-flop1/2
  Add1/1 -> If_Then_Else/2
  Unit_Delay3/1 -> Add1/2
  Logical Operator3/1 -> RS flip-flop1/1
  RS flip-flop1/2 -> Logical Operator2/1

== system EmE_MBD_Blockset/Logic and Bit Operations/D flip-flop with SR ==
  D : Inport
  CLK : Inport  Port=2
  !CLR : Inport  Port=3
  S : Inport  Port=4
  R : Inport  Port=5
  Enabled and Triggered Subsystem : Subsystem  TreatAsAtomicUnit=on
  If_Then_Else2 : $bdroot/Signal Routing/If_Then_Else
  If_Then_Else3 : $bdroot/Signal Routing/If_Then_Else
  Logical Operator1 : Logic  Operator=OR  OutDataTypeStr=boolean
  Q : Outport
  !Q : Outport  Port=2
  wires:
  !CLR/1 -> Enabled and Triggered Subsystem/Enable
  CLK/1 -> Enabled and Triggered Subsystem/Trigger
  Enabled and Triggered Subsystem/2(Out2) -> If_Then_Else3/3
  D/1 -> Enabled and Triggered Subsystem/1(In1)
  Enabled and Triggered Subsystem/1(Out1) -> If_Then_Else2/3
  If_Then_Else2/1 -> Q/1
  If_Then_Else3/1 -> !Q/1
  S/1 -> If_Then_Else2/2, Logical Operator1/1
  R/1 -> If_Then_Else3/2, Logical Operator1/2
  Logical Operator1/1 -> If_Then_Else3/1, If_Then_Else2/1

== system EmE_MBD_Blockset/Logic and Bit Operations/RS flip-flop ==
  Rp : Inport
  S : Inport  Port=2
  Logical Operator : Logic  OutDataTypeStr=boolean
  Logical Operator1 : Logic  Operator=OR  OutDataTypeStr=boolean
  Logical Operator2 : Logic  Operator=NOT  OutDataTypeStr=boolean
  Logical Operator3 : Logic  Operator=NOT  OutDataTypeStr=boolean
  Unit_Delay : UnitDelay  InitialCondition=false  SampleTime=-1
      settings: AttributesFormatString=IC: %<vinit>
  Q : Outport
  !Q : Outport  Port=2
  wires:
  Logical Operator3/1 -> Logical Operator/1
  Logical Operator1/1 -> Logical Operator/2
  S/1 -> Logical Operator1/1
  Rp/1 -> Logical Operator3/1
  Logical Operator/1 -> Q/1, Unit_Delay/1, Logical Operator2/1
  Unit_Delay/1 -> Logical Operator1/2
  Logical Operator2/1 -> !Q/1

== system EmE_MBD_Blockset/Logic and Bit Operations/SR flip-flop ==
  Sp : Inport
  R : Inport  Port=2
  Logical Operator : Logic  OutDataTypeStr=boolean
  Logical Operator1 : Logic  Operator=OR  OutDataTypeStr=boolean
  Logical Operator2 : Logic  Operator=NOT  OutDataTypeStr=boolean
  Logical Operator3 : Logic  Operator=NOT  OutDataTypeStr=boolean
  Unit_Delay : UnitDelay  InitialCondition=false  SampleTime=-1
      settings: AttributesFormatString=IC: %<vinit>
  Q : Outport
  !Q : Outport  Port=2
  wires:
  Logical Operator2/1 -> !Q/1
  Sp/1 -> Logical Operator1/1
  Logical Operator1/1 -> Q/1, Unit_Delay/1, Logical Operator2/1
  Logical Operator/1 -> Logical Operator1/2
  Logical Operator3/1 -> Logical Operator/1
  Unit_Delay/1 -> Logical Operator/2
  R/1 -> Logical Operator3/1

== system EmE_MBD_Blockset/Math Operators/Convert_polar_coordinates_to_rectangular_coordinates ==
  rho : Inport
  theta : Inport  Port=2
  Abs : $bdroot/Math Operators/Abs
  DEG_TO_RAD : $bdroot/Math Operators/Engineering_unit_conversion  eng_unit_type=angle  eng_unit_in=deg  eng_unit_out=rad  sat_on_int_overflow=off
  Product : Product  InputSameDT=on
  Product1 : Product  InputSameDT=on
  Trigonometric Function : Trigonometry  Operator=cos
  Trigonometric Function1 : Trigonometry
  x : Outport  LibraryBlock=$bdroot/Sinks/Out  OutputWhenDisabled=reset
  y : Outport  LibraryBlock=$bdroot/Sinks/Out  Port=2  OutputWhenDisabled=reset
  wires:
  theta/1 -> DEG_TO_RAD/1
  DEG_TO_RAD/1 -> Trigonometric Function/1, Trigonometric Function1/1
  rho/1 -> Abs/1
  Abs/1 -> Product1/1, Product/1
  Product1/1 -> y/1
  Product/1 -> x/1
  Trigonometric Function/1 -> Product/2
  Trigonometric Function1/1 -> Product1/2

== system EmE_MBD_Blockset/Math Operators/Convert_rectangular_coordinates_to_polar_coordinates ==
  x : Inport
  y : Inport  Port=2
  Math Function : Math  Operator=hypot  SaturateOnIntegerOverflow=on
  RAD_TO_DEG : $bdroot/Math Operators/Engineering_unit_conversion  eng_unit_type=angle  eng_unit_in=rad  eng_unit_out=deg  sat_on_int_overflow=off
  Trigonometric Function : Trigonometry  Operator=atan2
  rho : Outport  LibraryBlock=$bdroot/Sinks/Out  OutputWhenDisabled=reset
  theta : Outport  LibraryBlock=$bdroot/Sinks/Out  Port=2  OutputWhenDisabled=reset
  wires:
  RAD_TO_DEG/1 -> theta/1
  Trigonometric Function/1 -> RAD_TO_DEG/1
  Math Function/1 -> rho/1
  y/1 -> Math Function/2, Trigonometric Function/1
  x/1 -> Math Function/1, Trigonometric Function/2

== system EmE_MBD_Blockset/Math Operators/Convert_time ==
  In : Inport
  Constant : Constant  Value=1*60
  Data Type Conversion : DataTypeConversion
      settings: AttributesFormatString=%<OutDataTypeStr>
  Product1 : Product  InputSameDT=on
  Out : Outport  OutputWhenDisabled=reset
  wires:
  In/1 -> Data Type Conversion/1
  Product1/1 -> Out/1
  Data Type Conversion/1 -> Product1/1
  Constant/1 -> Product1/2

== system EmE_MBD_Blockset/Math Operators/Engineering_unit_conversion ==
  In : Inport
  Add : Sum  InputSameDT=on
  Data Type Conversion : $bdroot/Signal Attributes/Data Type Conversion  OutDataTypeStr=Inherit: Inherit via back propagation
  Gain_value : Constant  Value=0.73756
  Offset_value : Constant  Value=0
  Product : Product  InputSameDT=on
  Out : Outport  LibraryBlock=$bdroot/Sinks/Out  OutputWhenDisabled=reset
  wires:
  In/1 -> Data Type Conversion/1
  Product/1 -> Add/1
  Data Type Conversion/1 -> Product/1
  Gain_value/1 -> Product/2
  Add/1 -> Out/1
  Offset_value/1 -> Add/2

== system EmE_MBD_Blockset/Math Operators/Generic_linear_function ==
  X_value : Inport
  X1 : Inport  Port=2
  X2 : Inport  Port=3
  Y1 : Inport  Port=4
  Y2 : Inport  Port=5
  Add1 : Sum  InputSameDT=on
  Constant10 : Constant  Value=0.001
  Divide : Product  Inputs=*/  InputSameDT=on
  Dynamic_saturation2 : $bdroot/Discontinuities/Dynamic_saturation
  MinMax1 : MinMax  Inputs=2  InputSameDT=on
  MinMax2 : MinMax  Function=max  Inputs=2  InputSameDT=on
  MinMax3 : MinMax  Inputs=2  InputSameDT=on
  Product1 : Product  InputSameDT=on
  Subtract1 : Sum  Inputs=+-  InputSameDT=on
  Subtract2 : Sum  Inputs=+-  InputSameDT=on
  Subtract3 : Sum  Inputs=-+  InputSameDT=on
  Y_value : Outport
  wires:
  Dynamic_saturation2/1 -> Y_value/1
  Product1/1 -> Add1/1
  MinMax1/1 -> Divide/2
  Divide/1 -> Product1/1
  Add1/1 -> Dynamic_saturation2/2
  X_value/1 -> Subtract3/2
  Subtract3/1 -> Product1/2
  X1/1 -> Subtract2/2, Subtract3/1
  X2/1 -> Subtract2/1
  Y1/1 -> MinMax3/2, MinMax2/2, Add1/2, Subtract1/2
  Y2/1 -> Subtract1/1, MinMax3/1, MinMax2/1
  MinMax2/1 -> Dynamic_saturation2/1
  Subtract1/1 -> Divide/1
  Subtract2/1 -> MinMax1/1
  MinMax3/1 -> Dynamic_saturation2/3
  Constant10/1 -> MinMax1/2

== system EmE_MBD_Blockset/Math Operators/Min_max_index ==
  In2 : Inport
  Bus Creator : BusCreator  Inputs=1
  Find Nonzero Elements : Find  NumberOfInputDimensions=3
  MinMax : MinMax  Function=max  InputSameDT=on
  MinMax1 : MinMax  Function=max  InputSameDT=on
  Relational Operator : RelationalOperator  Operator===  OutDataTypeStr=boolean  RndMeth=Nearest  InputSameDT=on
  v : Outport  OutputWhenDisabled=reset
  i : Outport  Port=2  OutputWhenDisabled=reset
  wires:
  MinMax/1 -> i/1
  In2/1 -> Bus Creator/1
  Find Nonzero Elements/1 -> MinMax/1
  Bus Creator/1 -> MinMax1/1, Relational Operator/1
  Relational Operator/1 -> Find Nonzero Elements/1
  MinMax1/1 -> Relational Operator/2, v/1
